simulink model "vision_test"  (Simulink 7.6)
settings: Solver=FixedStepDiscrete  StartTime=0.0  StopTime=0  RelTol=1e-3
undefined symbols (not defined in the file or in its folder): gray, Rec, SDTV
libraries: vipconversions x4, vipsnks x2, vipsrcs x2, viptextngfix x2
settings Model: Creator=Administrator  LastModifiedBy=auvt
settings RTWCC: TargetLang=C++

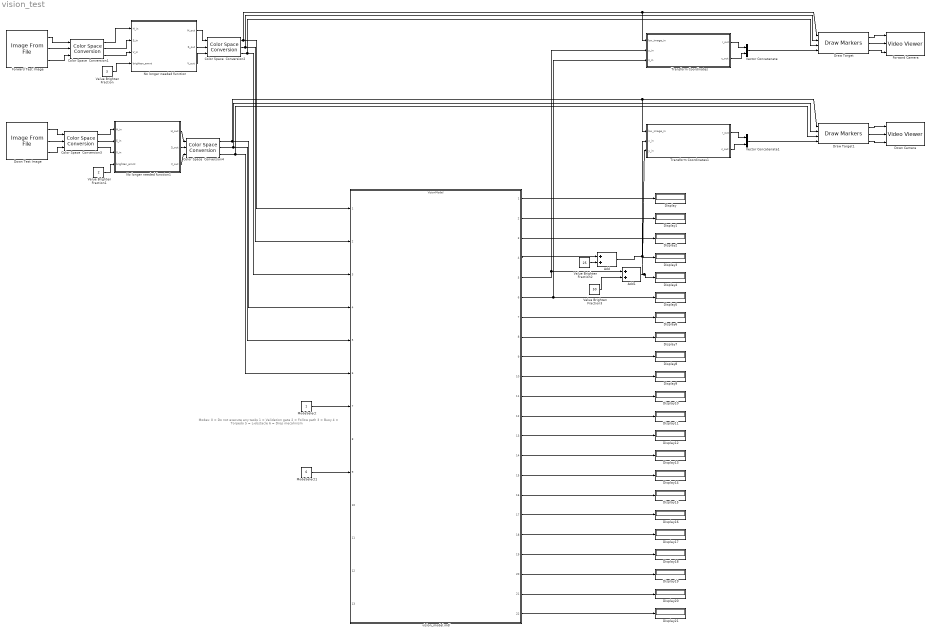
== system vision_test ==
  note: Modes:
      | 0 = Do not execute any tasks
      | 1 = Validation gate
      | 2 = Follow path
      | 3 = Buoy
      | 4 = Torpedo
      | 5 = L-obstacle
      | 6 = Drop mecahnism
  Add : Sum
  Add1 : Sum
  Color Space  Conversion1 : vipconversions/Color Space  Conversion  conversion=Obsolete  conversionActive=R'G'B' to HSV  wp_str=D50  rec=Rec. 601 (SDTV)  sys=1125/60/2:1  imagePorts=Separate color signals
  Color Space  Conversion2 : vipconversions/Color Space  Conversion  conversion=Obsolete  conversionActive=HSV to R'G'B'  wp_str=D50  rec=Rec. 601 (SDTV)  sys=1125/60/2:1  imagePorts=Separate color signals
  Color Space  Conversion3 : vipconversions/Color Space  Conversion  conversion=Obsolete  conversionActive=R'G'B' to HSV  wp_str=D50  rec=Rec. 601 (SDTV)  sys=1125/60/2:1  imagePorts=Separate color signals
  Color Space  Conversion4 : vipconversions/Color Space  Conversion  conversion=Obsolete  conversionActive=HSV to R'G'B'  wp_str=D50  rec=Rec. 601 (SDTV)  sys=1125/60/2:1  imagePorts=Separate color signals
  Display{,1..21} (22 alike) : Display
  Down Camera : vipsnks/Video Viewer  DialogControllerArgs=DataTag1  inputType=Obsolete7b  imagePorts=Separate color signals  useColorMap=off  colormapValue=gray(256)  specRange=off  minInputVal=0  maxInputVal=255  FigPos=[994 844 410 300]  AxisZoom=on  trueSizedOnce=off  OpenAtMdlStart=on
  Down Test Image : vipsrcs/Image From File  Tag=vipblks_nd  DialogController=vipDDGCreate  DialogControllerArgs=DataTag2  SystemSampleTime=-1  FileName=/home/auvt/auvc/src/vision/Modified_Files_for_Testing/Images/path9.bmp  imagePorts=Separate color signals  Ts=-1  ImageDataType=double  Signed=on  WordLength=16  sdImageDataType=uint(8)  FractionLengthMode=User-defined  FractionLength=15  OutPortLabels=R|G|B
  Draw Target : viptextngfix/Draw Markers  DialogController=vipDDGCreate  DialogControllerArgs=DataTag3  shape=X-mark  size=7  fill=off  fillClrSource=Specify via dialog  display=User-specified value  intensity=200  color=[0 0 0]  opacity=0.6  viewport=Entire image  antialiasing=off  inType=Obsolete  imagePorts=Separate color signals  prodOutputMode=Binary point scaling  prodOutputWordLength=32  prodOutputFracLength=14  memoryMode=Specify word length  memoryWordLength=16  memoryFracLength=15  roundingMode=Floor  overflowMode=off
  Draw Target1 : viptextngfix/Draw Markers  DialogController=vipDDGCreate  DialogControllerArgs=DataTag4  shape=X-mark  size=7  fill=off  fillClrSource=Specify via dialog  display=User-specified value  intensity=200  color=[0 0 0]  opacity=0.6  viewport=Entire image  antialiasing=off  inType=Obsolete  imagePorts=Separate color signals  prodOutputMode=Binary point scaling  prodOutputWordLength=32  prodOutputFracLength=14  memoryMode=Specify word length  memoryWordLength=16  memoryFracLength=15  roundingMode=Floor  overflowMode=off
  Forward Camera : vipsnks/Video Viewer  DialogControllerArgs=DataTag6  inputType=Obsolete7b  imagePorts=Separate color signals  useColorMap=off  colormapValue=gray(256)  specRange=off  minInputVal=0  maxInputVal=255  FigPos=[985 436 410 300]  AxisZoom=on  trueSizedOnce=off  OpenAtMdlStart=on
  Forward Test Image : vipsrcs/Image From File  Tag=vipblks_nd  DialogController=vipDDGCreate  DialogControllerArgs=DataTag7  SystemSampleTime=-1  FileName=/home/auvt/auvc/src/vision/Modified_Files_for_Testing/Images/gate13.bmp  imagePorts=Separate color signals  Ts=-1  ImageDataType=double  Signed=on  WordLength=16  sdImageDataType=uint(8)  FractionLengthMode=User-defined  FractionLength=15  OutPortLabels=R|G|B
  ModeSelect : Constant  SampleTime=-1
  ModeSelect1 : Constant  Value=6  SampleTime=-1
  No longer needed function : Stateflow chart  TreatAsAtomicUnit=on
  No longer needed function1 : Stateflow chart  TreatAsAtomicUnit=on
  Transform Coordinates : Stateflow chart  TreatAsAtomicUnit=on  SystemSampleTime=[1/30 0]
  Transform Coordinates1 : Stateflow chart  TreatAsAtomicUnit=on  SystemSampleTime=[1/30 0]
  Value Brighten Fraction : Constant  Value=3  SampleTime=-1
  Value Brighten Fraction1 : Constant  Value=2  SampleTime=-1
  Value Brighten Fraction2 : Constant  Value=25  SampleTime=-1
  Value Brighten Fraction3 : Constant  Value=50  SampleTime=-1
  Vector Concatenate : Concatenate  Mode=Multidimensional array
  Vector Concatenate1 : Concatenate  Mode=Multidimensional array
  vision_model.mdl : ModelReference  ModelNameDialog=VisionModel  SimulationMode=Accelerator  ModelReferenceVersion=1.405  CopyOfModelName=VisionModel
  wires:
  ModeSelect/1 -> vision_model.mdl/7
  vision_model.mdl/1 -> Display/1
  vision_model.mdl/2 -> Display1/1
  vision_model.mdl/3 -> Display2/1
  vision_model.mdl/5 -> Transform Coordinates/2(y_in), Add1/1
  vision_model.mdl/6 -> Display5/1, Transform Coordinates/3(z_in)
  vision_model.mdl/7 -> Display6/1
  vision_model.mdl/8 -> Display7/1
  vision_model.mdl/9 -> Display8/1
  vision_model.mdl/10 -> Display9/1
  vision_model.mdl/11 -> Display10/1
  vision_model.mdl/12 -> Display11/1
  vision_model.mdl/13 -> Display12/1
  vision_model.mdl/14 -> Display13/1
  vision_model.mdl/15 -> Display14/1
  vision_model.mdl/16 -> Display15/1
  vision_model.mdl/17 -> Display16/1
  vision_model.mdl/18 -> Display17/1
  Forward Test Image/2 -> Color Space  Conversion1/2
  Forward Test Image/1 -> Color Space  Conversion1/1
  Forward Test Image/3 -> Color Space  Conversion1/3
  Color Space  Conversion2/1 -> vision_model.mdl/1, Draw Target/1, Transform Coordinates/1(bw_image_in)
  Color Space  Conversion2/2 -> vision_model.mdl/2, Draw Target/2
  Color Space  Conversion2/3 -> vision_model.mdl/3, Draw Target/3
  Color Space  Conversion1/1 -> No longer needed function/1(H_in)
  Color Space  Conversion1/2 -> No longer needed function/2(S_in)
  Color Space  Conversion1/3 -> No longer needed function/3(V_in)
  No longer needed function/1(H_out) -> Color Space  Conversion2/1
  No longer needed function/2(S_out) -> Color Space  Conversion2/2
  No longer needed function/3(V_out) -> Color Space  Conversion2/3
  Value Brighten Fraction/1 -> No longer needed function/4(brighten_amnt)
  ModeSelect1/1 -> vision_model.mdl/9
  vision_model.mdl/19 -> Display18/1
  vision_model.mdl/20 -> Display19/1
  Vector Concatenate/1 -> Draw Target/4
  Draw Target/1 -> Forward Camera/1
  Draw Target/2 -> Forward Camera/2
  Draw Target/3 -> Forward Camera/3
  vision_model.mdl/21 -> Display20/1
  vision_model.mdl/22 -> Display21/1
  Transform Coordinates/1(r_out) -> Vector Concatenate/1
  Transform Coordinates/2(c_out) -> Vector Concatenate/2
  Draw Target1/1 -> Down Camera/1
  Draw Target1/2 -> Down Camera/2
  Transform Coordinates1/1(r_out) -> Vector Concatenate1/1
  Transform Coordinates1/2(c_out) -> Vector Concatenate1/2
  Draw Target1/3 -> Down Camera/3
  Vector Concatenate1/1 -> Draw Target1/4
  Color Space  Conversion3/1 -> No longer needed function1/1(H_in)
  Color Space  Conversion3/2 -> No longer needed function1/2(S_in)
  Color Space  Conversion3/3 -> No longer needed function1/3(V_in)
  No longer needed function1/1(H_out) -> Color Space  Conversion4/1
  No longer needed function1/2(S_out) -> Color Space  Conversion4/2
  No longer needed function1/3(V_out) -> Color Space  Conversion4/3
  Value Brighten Fraction1/1 -> No longer needed function1/4(brighten_amnt)
  Down Test Image/1 -> Color Space  Conversion3/1
  Down Test Image/2 -> Color Space  Conversion3/2
  Down Test Image/3 -> Color Space  Conversion3/3
  Color Space  Conversion4/1 -> vision_model.mdl/4, Draw Target1/1, Transform Coordinates1/1(bw_image_in)
  Color Space  Conversion4/2 -> vision_model.mdl/5, Draw Target1/2
  Color Space  Conversion4/3 -> vision_model.mdl/6, Draw Target1/3
  Value Brighten Fraction2/1 -> Add/2
  Value Brighten Fraction3/1 -> Add1/2
  vision_model.mdl/4 -> Add/1
  Add1/1 -> Display4/1, Transform Coordinates1/3(y_in)
  Add/1 -> Display3/1, Transform Coordinates1/2(x_in)

== matlab function No longer needed function ==
  data: H_in input double; S_in input double; V_in input double; H_out output double; S_out output double; V_out output double; brighten_amnt input double
function [H_out, S_out, V_out] = brightenImage(H_in, S_in, V_in, brighten_amnt)
%#eml


H_out = H_in;
S_out = S_in;
V_out = brighten_amnt.*V_in;




return

== matlab function Transform Coordinates ==
  data: bw_image_in input double; y_in input double; r_out output double; c_out output double; z_in input double
function [r_out, c_out] = transform_G2L_forward(bw_image_in, y_in, z_in)
% This function, "transform Global to Local coordinates," simply transforms
%   global coordinates that are sent to the controller into local
%   coordinates that can be displayed over images.
%
% 5-29-11

[rows, cols] = size(bw_image_in);
r_out = z_in + floor(rows/2);
c_out = y_in + floor(cols/2);

return

== matlab function Transform Coordinates1 ==
  data: bw_image_in input double; x_in input double; y_in input double; r_out output double; c_out output double
function [r_out, c_out] = transform_G2L_down(bw_image_in, x_in, y_in)
% This function, "transform Global to Local coordinates," simply transforms
%   global coordinates that are sent to the controller into local
%   coordinates that can be displayed over images.
%
% 5-29-11

[rows, cols] = size(bw_image_in);
r_out = -x_in + floor(rows/2);
c_out = y_in + floor(cols/2);

return

== matlab function No longer needed function1 ==
  data: H_in input double; S_in input double; V_in input double; H_out output double; S_out output double; V_out output double; brighten_amnt input double
function [H_out, S_out, V_out] = brightenImage(H_in, S_in, V_in, brighten_amnt)
%#eml


H_out = H_in;
S_out = S_in;
V_out = brighten_amnt.*V_in;




return
